simulink model "SCUTERacing_Model"  (R2020a)
settings: Solver=ode23tb  StartTime=0.0  StopTime=60  RelTol=5e-3
model workspace (MAT data in the model file):
  DLCXref = [0 8 9.5 18 34 34.5 45 50 60]
  DLCYref = [0 0 -4.5 -4 -3.75 1.5 0.5 0 0]
  VEH : object (value not decoded)
  extRef = 0.01
  mot : object (value not decoded)
symbols that are objects in the model workspace (value not decoded): mot, VEH
undefined symbols (not defined in the file or in its folder): Batt, h, Right
libraries: simulink x6, vehdynlibscenariocommon x4, sim3dlib x2, vehdynlibdriver x1, autolibshared x1, vehdynlibviscommon x1
(part 2 of 2)

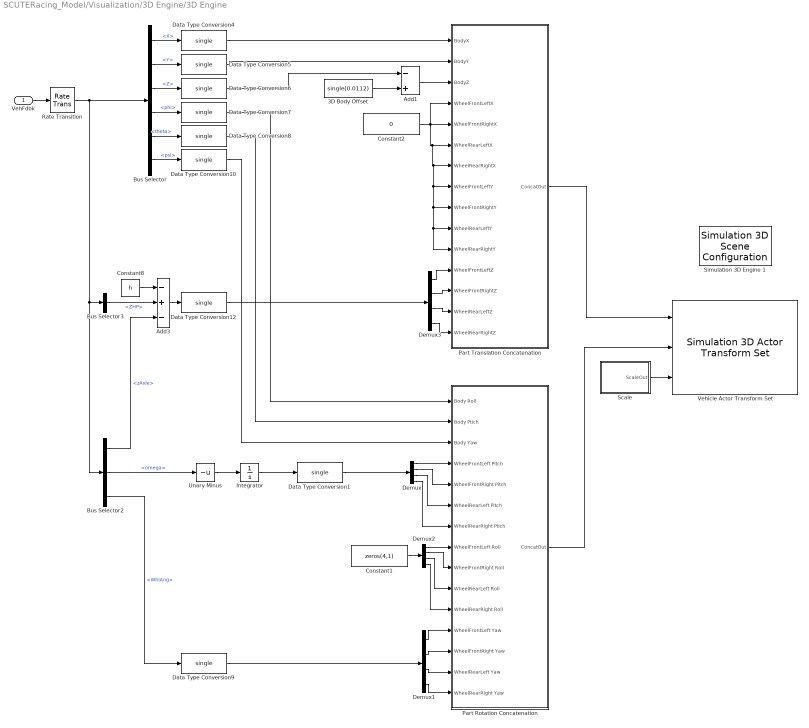
== system SCUTERacing_Model/Visualization/3D Engine/3D Engine ==
  VehFdbk : Inport
  3D Body Offset : Constant  Value=single(0.0112)  OutDataTypeStr=single
  Add1 : Sum  Inputs=-+
  Add3 : Sum  Inputs=-+-
  Bus Selector : BusSelector  OutputSignals=Body.X,Body.Y,Body.Z,Body.phi,Body.theta,Body.psi
  Bus Selector2 : BusSelector  OutputSignals=Wheels.zAxle,Wheels.omega,Driveline.WhlAng
  Bus Selector3 : BusSelector  OutputSignals=Body.ZHP
  Constant1 : Constant  Value=zeros(4,1)  OutDataTypeStr=single
  Constant2 : Constant  Value=0  OutDataTypeStr=single
  Constant8 : Constant  Value=h
  Data Type Conversion{1,4..10,12} (9 alike) : DataTypeConversion  OutDataTypeStr=single
  Demux{,1..3} (4 alike) : Demux
  Integrator : Integrator  WrapState=on  WrappedStateUpperValue=2*pi  WrappedStateLowerValue=0  ZeroCross=off
  Part Rotation Concatenation : Subsystem
  Part Translation Concatenation : Subsystem
  Rate Transition : RateTransition  OutPortSampleTime=dt3D
  Scale : Subsystem
  Simulation 3D Engine 1 : sim3dlib/Simulation 3D Scene Configuration  Priority=1  ProjectFormat=Default Scenes  SceneDesc=Straight road  ProjectName=VehicleSimulation.exe  ScenePath=/Game/Maps/HwStrght  vehTagList={'Scene Origin'}  vehTag=Scene Origin  OpVisEn=off  Ts=dt3D  EnableWindow=on  sensorTag=MainCamera1  sensorId=1  sensorName=MainCamera1  mountLoc=Origin  offsetFlag=off  tmountOffset=[0, 0, 0]  rmountOffset=[0, 0, 0]  HorizontalResolution=1280  VerticalResolution=720  HorizontalFOV=60  mountPoint=[0 0 0]  mountOrientation=[0 0 0]  aMode=aMode  ID=1
      settings: AttributesFormatString=Priority: %<Priority>  SourceProductBaseCode=DR,VE
  Unary Minus : UnaryMinus
  Vehicle Actor Transform Set : sim3dlib/Simulation 3D Actor Transform Set  ActorTag=SimulinkVehicle1  ActorType=Passenger vehicle  PassVehMesh=Muscle car  VehColor=Red  NumberOfParts=5  CustNumOfParts=3  Translation=[0 0 1; 0 0 0; 0 0 0; 0 0 0; 0 0 0]  Rotation=[0 0 0; 0 0 0; 0 0 0; 0 0 0; 0 0 0]  Scale=[1 1 1; 1 1 1; 1 1 1; 1 1 1; 1 1 1]  Ts=dt3D
      settings: SourceProductBaseCode=DR,VE
  wires:
  Unary Minus/1 -> Integrator/1
  Bus Selector3/1 -> Add3/2  "<ZHP>"
  Add3/1 -> Data Type Conversion12/1
  Bus Selector2/1 -> Add3/3  "<zAxle>"
  Constant8/1 -> Add3/1
  Rate Transition/1 -> Bus Selector/1, Bus Selector3/1, Bus Selector2/1
  Scale/1(ScaleOut) -> Vehicle Actor Transform Set/3
  Demux/4 -> Part Rotation Concatenation/7(WheelRearRight Ptich)
  Demux/3 -> Part Rotation Concatenation/6(WheelRearLeft Pitch)
  Demux/2 -> Part Rotation Concatenation/5(WheelFrontRight Pitch)
  Demux/1 -> Part Rotation Concatenation/4(WheelFrontLeft Pitch)
  Constant1/1 -> Demux2/1
  Bus Selector/4 -> Data Type Conversion7/1  "<phi>"
  Data Type Conversion6/1 -> Add1/1
  Part Rotation Concatenation/1(ConcatOut) -> Vehicle Actor Transform Set/2
  Part Translation Concatenation/1(ConcatOut) -> Vehicle Actor Transform Set/1
  Data Type Conversion12/1 -> Demux3/1
  Demux3/4 -> Part Translation Concatenation/15(WheelRearRightZ)
  Demux3/3 -> Part Translation Concatenation/14(WheelRearLeftZ)
  Demux3/1 -> Part Translation Concatenation/12(WheelFrontLeftZ)
  Demux3/2 -> Part Translation Concatenation/13(WheelFrontRightZ)
  VehFdbk/1 -> Rate Transition/1
  Add1/1 -> Part Translation Concatenation/3(BodyZ)
  3D Body Offset/1 -> Add1/2
  Demux1/4 -> Part Rotation Concatenation/15(WheelRearRight Yaw)
  Demux1/3 -> Part Rotation Concatenation/14(WheelRearLeft Yaw)
  Demux2/1 -> Part Rotation Concatenation/8(WheelFrontLeft Roll)
  Demux2/2 -> Part Rotation Concatenation/9(WheelFrontRight Roll)
  Demux2/3 -> Part Rotation Concatenation/10(WheelRearLeft Roll)
  Demux2/4 -> Part Rotation Concatenation/11(WheelRearRight Roll)
  Bus Selector2/3 -> Data Type Conversion9/1  "<WhlAng>"
  Bus Selector2/2 -> Unary Minus/1  "<omega>"
  Data Type Conversion9/1 -> Demux1/1
  Demux1/1 -> Part Rotation Concatenation/12(WheelFrontLeft Yaw)
  Demux1/2 -> Part Rotation Concatenation/13(WheelFrontRight Yaw)
  Integrator/1 -> Data Type Conversion1/1
  Data Type Conversion1/1 -> Demux/1
  Data Type Conversion8/1 -> Part Rotation Concatenation/2(Body Ptich)
  Data Type Conversion5/1 -> Part Translation Concatenation/2(BodyY)
  Data Type Conversion10/1 -> Part Rotation Concatenation/3(Body Yaw)
  Constant2/1 -> Part Translation Concatenation/5(WheelFrontRightX), Part Translation Concatenation/6(WheelRearLeftX), Part Translation Concatenation/7(WheelRearRightX), Part Translation Concatenation/8(WheelFrontLeftY), Part Translation Concatenation/9(WheelFrontRightY), Part Translation Concatenation/10(WheelRearLeftY), Part Translation Concatenation/11(WheelRearRightY), Part Translation Concatenation/4(WheelFrontLeftX)
  Data Type Conversion4/1 -> Part Translation Concatenation/1(BodyX)
  Data Type Conversion7/1 -> Part Rotation Concatenation/1(Body Roll)
  Bus Selector/1 -> Data Type Conversion4/1  "<X>"
  Bus Selector/2 -> Data Type Conversion5/1  "<Y>"
  Bus Selector/3 -> Data Type Conversion6/1  "<Z>"
  Bus Selector/6 -> Data Type Conversion10/1  "<psi>"
  Bus Selector/5 -> Data Type Conversion8/1  "<theta>"

== system SCUTERacing_Model/Visualization/3D Engine/3D Engine Disabled ==
  VehFdbk : Inport
  Terminator : Terminator
  wires:
  VehFdbk/1 -> Terminator/1

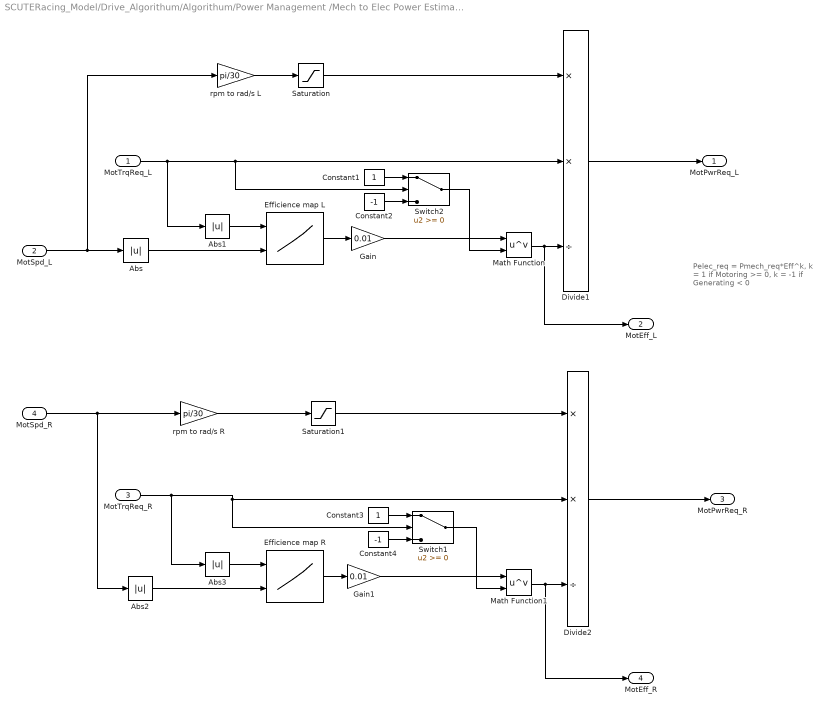
== system SCUTERacing_Model/Drive_Algorithum/Algorithum/Power Management /Mech to Elec Power Estimate ==
  note: Pelec_req = Pmech_req*Eff^k,
      | k = 1 if Motoring >= 0,
      | k = -1 if Generating < 0
  MotTrqReq_L : Inport
  MotSpd_L : Inport  Port=2
  MotTrqReq_R : Inport  Port=3
  MotSpd_R : Inport  Port=4
  Abs{,1..3} (4 alike) : Abs
  Constant1 : Constant  SampleTime=-1
  Constant2 : Constant  Value=-1  SampleTime=-1
  Constant3 : Constant  SampleTime=-1
  Constant4 : Constant  Value=-1  SampleTime=-1
  Divide1 : Product  Inputs=**/
  Divide2 : Product  Inputs=**/
  Efficience map L : Lookup_n-D  BreakpointsForDimension1=mot.mapL.trqindex  BreakpointsForDimension2=mot.mapL.spdindex  BeginIndexSearchUsingPreviousIndexResult=on  Table=mot.mapL.eff  ExtrapMethod=Clip  UseLastTableValue=on  InternalRulePriority=Speed  OutDataTypeStr=Inherit: Inherit from 'Table data'  RndMeth=Simplest  InputSameDT=on
  Efficience map R : Lookup_n-D  BreakpointsForDimension1=mot.mapR.trqindex  BreakpointsForDimension2=mot.mapR.spdindex  BeginIndexSearchUsingPreviousIndexResult=on  Table=mot.mapR.eff  ExtrapMethod=Clip  UseLastTableValue=on  InternalRulePriority=Speed  OutDataTypeStr=Inherit: Inherit from 'Table data'  RndMeth=Simplest  InputSameDT=on
  Gain : Gain  Gain=0.01
  Gain1 : Gain  Gain=0.01
  Math Function : Math  Operator=pow  SignedPower=on  OutputSignalType=real  SaturateOnIntegerOverflow=on
  Math Function1 : Math  Operator=pow  SignedPower=on  OutputSignalType=real  SaturateOnIntegerOverflow=on
  Saturation : Saturate  UpperLimit=inf  LowerLimit=10
  Saturation1 : Saturate  UpperLimit=inf  LowerLimit=10
  Switch1 : Switch
  Switch2 : Switch
  rpm to rad/s L : Gain  Gain=pi/30
  rpm to rad/s R : Gain  Gain=pi/30
  MotPwrReq_L : Outport  VectorParamsAs1DForOutWhenUnconnected=off
  MotEff_L : Outport  Port=2  VectorParamsAs1DForOutWhenUnconnected=off
  MotPwrReq_R : Outport  Port=3  VectorParamsAs1DForOutWhenUnconnected=off
  MotEff_R : Outport  Port=4  VectorParamsAs1DForOutWhenUnconnected=off
  wires:
  rpm to rad/s L/1 -> Saturation/1
  MotSpd_R/1 -> Abs2/1, rpm to rad/s R/1
  MotTrqReq_R/1 -> Switch1/2, Divide2/2, Abs3/1
  MotSpd_L/1 -> rpm to rad/s L/1, Abs/1
  Saturation/1 -> Divide1/1
  Saturation1/1 -> Divide2/1
  Efficience map R/1 -> Gain1/1
  Efficience map L/1 -> Gain/1
  MotTrqReq_L/1 -> Divide1/2, Switch2/2, Abs1/1
  rpm to rad/s R/1 -> Saturation1/1
  Divide1/1 -> MotPwrReq_L/1
  Divide2/1 -> MotPwrReq_R/1
  Abs/1 -> Efficience map L/2
  Abs1/1 -> Efficience map L/1
  Abs2/1 -> Efficience map R/2
  Abs3/1 -> Efficience map R/1
  Gain/1 -> Math Function/1
  Constant2/1 -> Switch2/3
  Constant1/1 -> Switch2/1
  Math Function/1 -> MotEff_L/1, Divide1/3
  Switch2/1 -> Math Function/2
  Switch1/1 -> Math Function1/2
  Constant3/1 -> Switch1/1
  Constant4/1 -> Switch1/3
  Math Function1/1 -> MotEff_R/1, Divide2/3
  Gain1/1 -> Math Function1/1

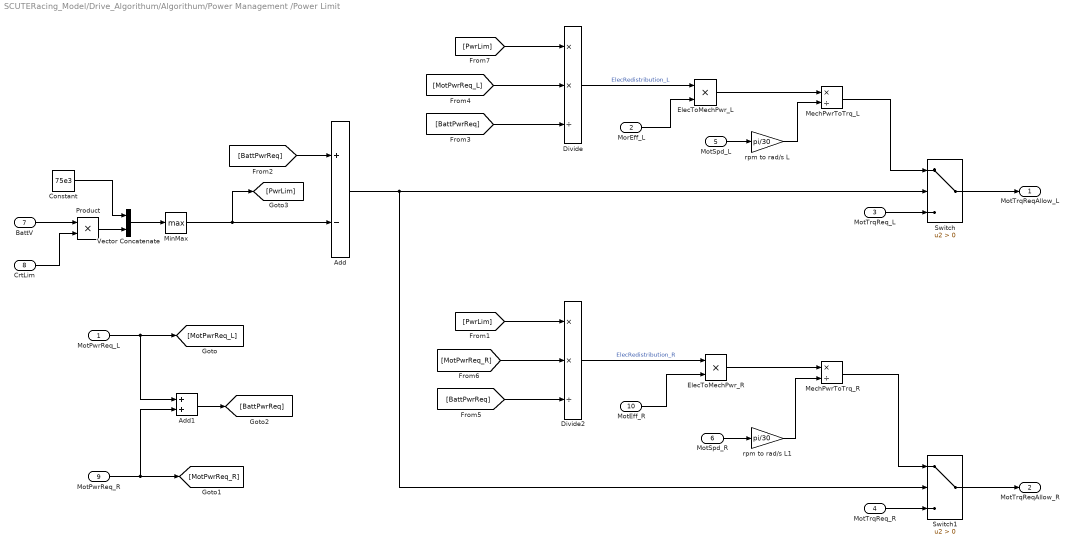
== system SCUTERacing_Model/Drive_Algorithum/Algorithum/Power Management /Power Limit ==
  MotPwrReq_L : Inport
  MorEff_L : Inport  Port=2
  MotTrqReq_L : Inport  Port=3
  MotTrqReq_R : Inport  Port=4
  MotSpd_L : Inport  Port=5
  MotSpd_R : Inport  Port=6
  BattV : Inport  Port=7
  CrtLim : Inport  Port=8
  MotPwrReq_R : Inport  Port=9
  MotEff_R : Inport  Port=10
  Add : Sum  Inputs=+-
  Add1 : Sum
  Constant : Constant  Value=75e3
  Divide : Product  Inputs=**/
  Divide2 : Product  Inputs=**/
  ElecToMechPwr_L : Product  Inputs=**
  ElecToMechPwr_R : Product  Inputs=**
  MechPwrToTrq_L : Product  Inputs=*/
  MechPwrToTrq_R : Product  Inputs=*/
  MinMax : MinMax  Function=max
  Product : Product
  Switch : Switch  Criteria=u2 > Threshold
  Switch1 : Switch  Criteria=u2 > Threshold
  Vector Concatenate : Concatenate
  rpm to rad/s L : Gain  Gain=pi/30
  rpm to rad/s L1 : Gain  Gain=pi/30
  MotTrqReqAllow_L : Outport  VectorParamsAs1DForOutWhenUnconnected=off
  MotTrqReqAllow_R : Outport  Port=2  VectorParamsAs1DForOutWhenUnconnected=off
  wires:
  Add/1 -> Switch1/2, Switch/2
  MotPwrReq_L/1 -> Add1/1, [MotPwrReq_L]
  MotPwrReq_R/1 -> Add1/2, [MotPwrReq_R]
  Add1/1 -> [BattPwrReq]
  [BattPwrReq] -> Add/1
  Switch/1 -> MotTrqReqAllow_L/1
  Switch1/1 -> MotTrqReqAllow_R/1
  [BattPwrReq] -> Divide2/3
  [MotPwrReq_R] -> Divide2/2
  [PwrLim] -> Divide/1
  [BattPwrReq] -> Divide/3
  [MotPwrReq_L] -> Divide/2
  MotTrqReq_L/1 -> Switch/3
  [PwrLim] -> Divide2/1
  MotTrqReq_R/1 -> Switch1/3
  BattV/1 -> Product/1
  CrtLim/1 -> Product/2
  MinMax/1 -> Add/2, [PwrLim]
  Product/1 -> Vector Concatenate/2
  Vector Concatenate/1 -> MinMax/1
  Constant/1 -> Vector Concatenate/1
  Divide/1 -> ElecToMechPwr_L/1  "ElecRedistribution_L"
  MorEff_L/1 -> ElecToMechPwr_L/2
  ElecToMechPwr_L/1 -> MechPwrToTrq_L/1
  MotSpd_L/1 -> rpm to rad/s L/1
  rpm to rad/s L/1 -> MechPwrToTrq_L/2
  MechPwrToTrq_L/1 -> Switch/1
  Divide2/1 -> ElecToMechPwr_R/1  "ElecRedistribution_R"
  MotEff_R/1 -> ElecToMechPwr_R/2
  MotSpd_R/1 -> rpm to rad/s L1/1
  ElecToMechPwr_R/1 -> MechPwrToTrq_R/1
  rpm to rad/s L1/1 -> MechPwrToTrq_R/2
  MechPwrToTrq_R/1 -> Switch1/1

== system SCUTERacing_Model/Drive_Algorithum/Algorithum/Power Management /Regen Power Limit ==
  MotTrqCmdRegen_L : Inport
  MotTrqCmdRegen_R : Inport  Port=2
  "BattSoc " : Inport  Port=3
  BrkCmd : Inport  Port=4
  MotSpd_L : Inport  Port=5
  MotSpd_R : Inport  Port=6
  ChrgLmt : Lookup_n-D  NumberOfTableDimensions=1  BreakpointsForDimension1=Batt.Limit.SOC  Table=Batt.Limit.Charge  ExtrapMethod=Clip  UseLastTableValue=on  InternalRulePriority=Speed  RndMeth=Simplest  InputSameDT=on
  Constant1 : Constant  Value=0
  Divide : Product  Inputs=/**
  Efficience map L1 : Lookup_n-D  BreakpointsForDimension1=mot.mapL.trqindex  BreakpointsForDimension2=mot.mapL.spdindex  BeginIndexSearchUsingPreviousIndexResult=on  Table=mot.mapL.eff  ExtrapMethod=Clip  UseLastTableValue=on  InternalRulePriority=Speed  OutDataTypeStr=Inherit: Inherit from 'Table data'  RndMeth=Simplest  InputSameDT=on
  Gain4 : Gain  Gain=-1
  MaxChrg : Constant  Value=-380*30
  Product : Product
  Saturation Dynamic : simulink/Discontinuities/Saturation Dynamic  OutMin=[]  OutMax=[]  OutDataTypeStr=Inherit: Same as second input  OutDataType=fixdt(1, 16)  OutScaling=2^-10  DoSatur=off
  Saturation2 : Saturate  UpperLimit=inf  LowerLimit=10
  rpm to rad/s L1 : Gain  Gain=pi/30
  MotTrqCmdRegenAllow_L : Outport  VectorParamsAs1DForOutWhenUnconnected=off
  MotTrqCmdRegenAllow_R : Outport  Port=2  VectorParamsAs1DForOutWhenUnconnected=off
  wires:
  Efficience map L1/1 -> Divide/1
  ? -> ChrgLmt/1
  Saturation2/1 -> Divide/2
  Saturation Dynamic/1 -> ?
  rpm to rad/s L1/1 -> Saturation2/1
  ChrgLmt/1 -> Product/1
  Constant1/1 -> Saturation Dynamic/1
  Divide/1 -> Saturation Dynamic/2
  MaxChrg/1 -> Product/2
  ? -> rpm to rad/s L1/1, Efficience map L1/2
  Gain4/1 -> Divide/3
  Product/1 -> Saturation Dynamic/3
  ? -> Efficience map L1/1, Gain4/1

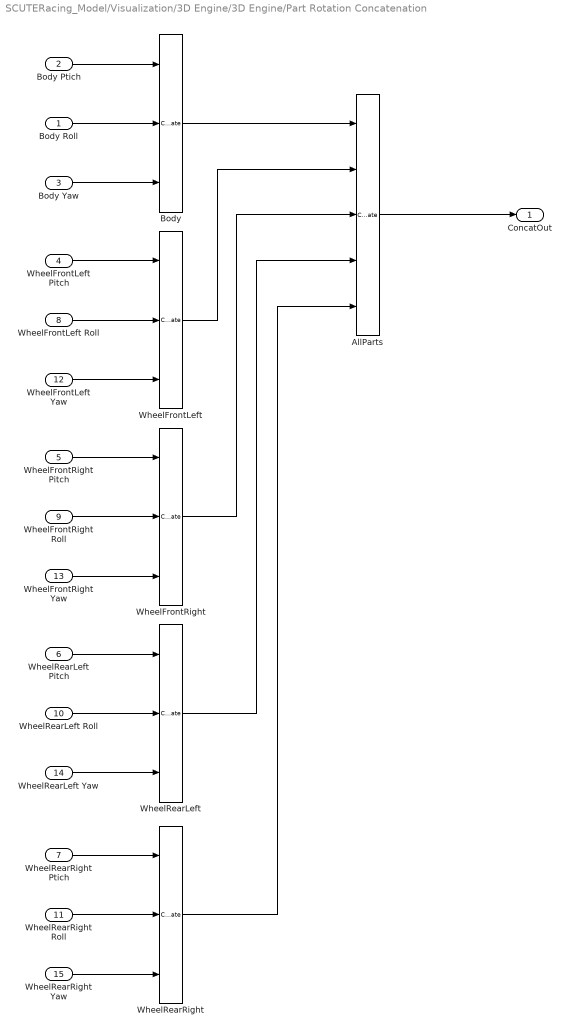
== system SCUTERacing_Model/Visualization/3D Engine/3D Engine/Part Rotation Concatenation ==
  Body Roll : Inport
  Body Ptich : Inport  Port=2
  Body Yaw : Inport  Port=3
  WheelFrontLeft Pitch : Inport  Port=4
  WheelFrontRight Pitch : Inport  Port=5
  WheelRearLeft Pitch : Inport  Port=6
  WheelRearRight Ptich : Inport  Port=7
  WheelFrontLeft Roll : Inport  Port=8
  WheelFrontRight Roll : Inport  Port=9
  WheelRearLeft Roll : Inport  Port=10
  WheelRearRight Roll : Inport  Port=11
  WheelFrontLeft Yaw : Inport  Port=12
  WheelFrontRight Yaw : Inport  Port=13
  WheelRearLeft Yaw : Inport  Port=14
  WheelRearRight Yaw : Inport  Port=15
  AllParts : Concatenate  NumInputs=5  Mode=Multidimensional array
  Body : Concatenate  NumInputs=3  Mode=Multidimensional array  ConcatenateDimension=2
  WheelFrontLeft : Concatenate  NumInputs=3  Mode=Multidimensional array  ConcatenateDimension=2
  WheelFrontRight : Concatenate  NumInputs=3  Mode=Multidimensional array  ConcatenateDimension=2
  WheelRearLeft : Concatenate  NumInputs=3  Mode=Multidimensional array  ConcatenateDimension=2
  WheelRearRight : Concatenate  NumInputs=3  Mode=Multidimensional array  ConcatenateDimension=2
  ConcatOut : Outport  VectorParamsAs1DForOutWhenUnconnected=off
  wires:
  Body Ptich/1 -> Body/1
  Body Yaw/1 -> Body/3
  WheelFrontLeft Pitch/1 -> WheelFrontLeft/1
  WheelFrontLeft Yaw/1 -> WheelFrontLeft/3
  WheelFrontLeft Roll/1 -> WheelFrontLeft/2
  Body Roll/1 -> Body/2
  WheelFrontLeft/1 -> AllParts/2
  WheelRearRight Ptich/1 -> WheelRearRight/1
  Body/1 -> AllParts/1
  WheelRearLeft/1 -> AllParts/4
  WheelFrontRight/1 -> AllParts/3
  WheelRearRight Yaw/1 -> WheelRearRight/3
  WheelFrontRight Roll/1 -> WheelFrontRight/2
  WheelFrontRight Pitch/1 -> WheelFrontRight/1
  WheelRearRight Roll/1 -> WheelRearRight/2
  WheelRearLeft Yaw/1 -> WheelRearLeft/3
  AllParts/1 -> ConcatOut/1
  WheelRearLeft Roll/1 -> WheelRearLeft/2
  WheelRearRight/1 -> AllParts/5
  WheelRearLeft Pitch/1 -> WheelRearLeft/1
  WheelFrontRight Yaw/1 -> WheelFrontRight/3

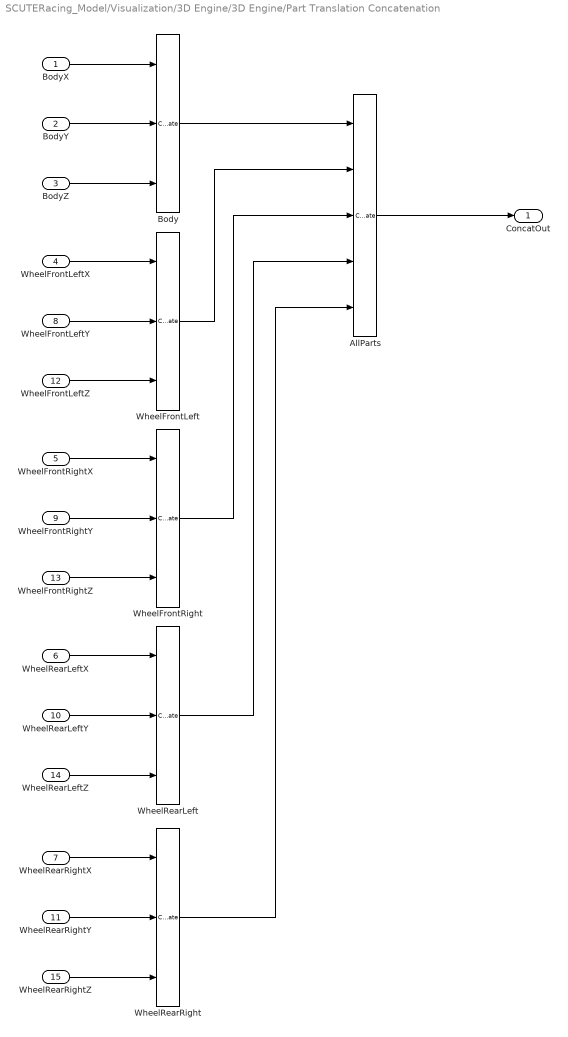
== system SCUTERacing_Model/Visualization/3D Engine/3D Engine/Part Translation Concatenation ==
  BodyX : Inport
  BodyY : Inport  Port=2
  BodyZ : Inport  Port=3
  WheelFrontLeftX : Inport  Port=4
  WheelFrontRightX : Inport  Port=5
  WheelRearLeftX : Inport  Port=6
  WheelRearRightX : Inport  Port=7
  WheelFrontLeftY : Inport  Port=8
  WheelFrontRightY : Inport  Port=9
  WheelRearLeftY : Inport  Port=10
  WheelRearRightY : Inport  Port=11
  WheelFrontLeftZ : Inport  Port=12
  WheelFrontRightZ : Inport  Port=13
  WheelRearLeftZ : Inport  Port=14
  WheelRearRightZ : Inport  Port=15
  AllParts : Concatenate  NumInputs=5  Mode=Multidimensional array
  Body : Concatenate  NumInputs=3  Mode=Multidimensional array  ConcatenateDimension=2
  WheelFrontLeft : Concatenate  NumInputs=3  Mode=Multidimensional array  ConcatenateDimension=2
  WheelFrontRight : Concatenate  NumInputs=3  Mode=Multidimensional array  ConcatenateDimension=2
  WheelRearLeft : Concatenate  NumInputs=3  Mode=Multidimensional array  ConcatenateDimension=2
  WheelRearRight : Concatenate  NumInputs=3  Mode=Multidimensional array  ConcatenateDimension=2
  ConcatOut : Outport  VectorParamsAs1DForOutWhenUnconnected=off
  wires:
  BodyX/1 -> Body/1
  BodyZ/1 -> Body/3
  WheelFrontLeftX/1 -> WheelFrontLeft/1
  WheelFrontLeftZ/1 -> WheelFrontLeft/3
  WheelFrontLeftY/1 -> WheelFrontLeft/2
  BodyY/1 -> Body/2
  WheelFrontLeft/1 -> AllParts/2
  WheelRearRightX/1 -> WheelRearRight/1
  Body/1 -> AllParts/1
  WheelRearLeft/1 -> AllParts/4
  WheelFrontRight/1 -> AllParts/3
  WheelRearRightZ/1 -> WheelRearRight/3
  WheelFrontRightY/1 -> WheelFrontRight/2
  WheelFrontRightX/1 -> WheelFrontRight/1
  WheelRearRightY/1 -> WheelRearRight/2
  WheelRearLeftZ/1 -> WheelRearLeft/3
  AllParts/1 -> ConcatOut/1
  WheelRearLeftY/1 -> WheelRearLeft/2
  WheelRearRight/1 -> AllParts/5
  WheelRearLeftX/1 -> WheelRearLeft/1
  WheelFrontRightZ/1 -> WheelFrontRight/3

== system SCUTERacing_Model/Visualization/3D Engine/3D Engine/Scale ==
  Constant{1..12,17,32..33} (15 alike) : Constant  OutDataTypeStr=single
  PartConcatenation : Subsystem
  ScaleOut : Outport  VectorParamsAs1DForOutWhenUnconnected=off
  wires:
  Constant10/1 -> PartConcatenation/15(WheelRearRightZ)
  Constant9/1 -> PartConcatenation/14(WheelRearRightY)
  Constant11/1 -> PartConcatenation/13(WheelRearRightX)
  Constant7/1 -> PartConcatenation/12(WheelRearLeftZ)
  Constant6/1 -> PartConcatenation/11(WheelRearLeftY)
  Constant8/1 -> PartConcatenation/10(WheelRearLeftX)
  Constant4/1 -> PartConcatenation/9(WheelFrontRightZ)
  Constant3/1 -> PartConcatenation/8(WheelFrontRightY)
  Constant5/1 -> PartConcatenation/7(WheelFrontRightX)
  Constant2/1 -> PartConcatenation/6(WheelFrontLeftZ)
  Constant1/1 -> PartConcatenation/5(WheelFrontLeftY)
  Constant33/1 -> PartConcatenation/4(WheelFrontLeftX)
  Constant32/1 -> PartConcatenation/3(BodyZ)
  Constant17/1 -> PartConcatenation/2(BodyY)
  Constant12/1 -> PartConcatenation/1(BodyX)
  PartConcatenation/1(ConcatOut) -> ScaleOut/1

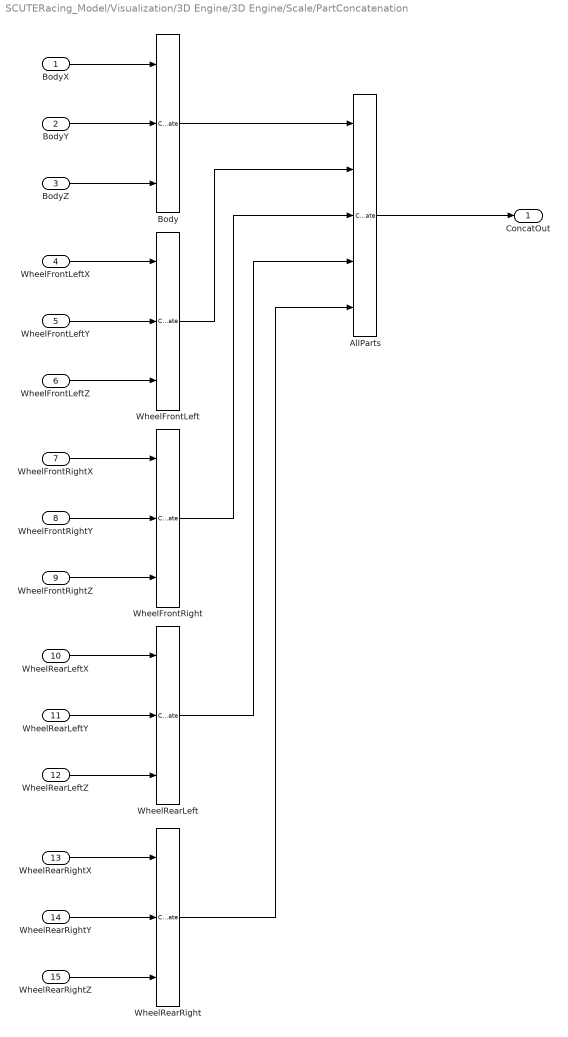
== system SCUTERacing_Model/Visualization/3D Engine/3D Engine/Scale/PartConcatenation ==
  BodyX : Inport
  BodyY : Inport  Port=2
  BodyZ : Inport  Port=3
  WheelFrontLeftX : Inport  Port=4
  WheelFrontLeftY : Inport  Port=5
  WheelFrontLeftZ : Inport  Port=6
  WheelFrontRightX : Inport  Port=7
  WheelFrontRightY : Inport  Port=8
  WheelFrontRightZ : Inport  Port=9
  WheelRearLeftX : Inport  Port=10
  WheelRearLeftY : Inport  Port=11
  WheelRearLeftZ : Inport  Port=12
  WheelRearRightX : Inport  Port=13
  WheelRearRightY : Inport  Port=14
  WheelRearRightZ : Inport  Port=15
  AllParts : Concatenate  NumInputs=5  Mode=Multidimensional array
  Body : Concatenate  NumInputs=3  Mode=Multidimensional array  ConcatenateDimension=2
  WheelFrontLeft : Concatenate  NumInputs=3  Mode=Multidimensional array  ConcatenateDimension=2
  WheelFrontRight : Concatenate  NumInputs=3  Mode=Multidimensional array  ConcatenateDimension=2
  WheelRearLeft : Concatenate  NumInputs=3  Mode=Multidimensional array  ConcatenateDimension=2
  WheelRearRight : Concatenate  NumInputs=3  Mode=Multidimensional array  ConcatenateDimension=2
  ConcatOut : Outport  VectorParamsAs1DForOutWhenUnconnected=off
  wires:
  BodyX/1 -> Body/1
  BodyZ/1 -> Body/3
  WheelFrontLeftX/1 -> WheelFrontLeft/1
  WheelFrontLeftZ/1 -> WheelFrontLeft/3
  WheelFrontLeftY/1 -> WheelFrontLeft/2
  BodyY/1 -> Body/2
  WheelFrontLeft/1 -> AllParts/2
  WheelRearRightX/1 -> WheelRearRight/1
  Body/1 -> AllParts/1
  WheelRearLeft/1 -> AllParts/4
  WheelFrontRight/1 -> AllParts/3
  WheelRearRightZ/1 -> WheelRearRight/3
  WheelFrontRightY/1 -> WheelFrontRight/2
  WheelFrontRightX/1 -> WheelFrontRight/1
  WheelRearRightY/1 -> WheelRearRight/2
  WheelRearLeftZ/1 -> WheelRearLeft/3
  AllParts/1 -> ConcatOut/1
  WheelRearLeftY/1 -> WheelRearLeft/2
  WheelRearRight/1 -> AllParts/5
  WheelRearLeftX/1 -> WheelRearLeft/1
  WheelFrontRightZ/1 -> WheelFrontRight/3

== matlab function SCUTERacing_Model/Reference Generator/Constant Radius/Constant Radius/MATLAB Function ==
  data: yRef output; Rref input; VehRef output size=3; InertCGDisp input; Xo input; Yo input; psio input; turnDirMask parameter
function [yRef,VehRef] = fcn(Rref, InertCGDisp,Xo,Yo,psio,turnDirMask)
if turnDirMask==1
    turnDir = 1;
else
    turnDir = -1;
end
Xo=Xo+Rref*sin(psio).*turnDir;
Yo=Yo-Rref*cos(psio).*turnDir;
RVeh = sqrt((InertCGDisp(1)-Xo).^2+(InertCGDisp(2)-Yo).^2);
theta = atan2(InertCGDisp(1)-Xo,InertCGDisp(2)-Yo)+atan2(0*2,RVeh).*turnDir;
VehRefX = Rref*sin(theta)+Xo;
VehRefY = Rref*cos(theta)+Yo;
VehRef = [VehRefX; VehRefY;InertCGDisp(3)];
yRef=-(Rref-RVeh).*turnDir;
% Rref = Rref.*turnDir;
% RVeh= RVeh.*turnDir;
